simulink model "Drone_Response_v5"  (R2024b)
settings: Solver=VariableStepAuto  StartTime=0.0  StopTime=17.980265000000003  MaxStep=0.01  RelTol=1e-6  AbsTol=1e-8
model workspace (MAT data in the model file):
  Fx_gust = 1
  Fy_gust = 1
  Fz_gust = 0.5
  Ixx = 0.05
  Iyy = 0.05
  Izz = 0.1
  Kd_phi = 0.5
  Kd_psi = 0.12
  Kd_theta = 0.28
  Kd_x = 0.5
  Kd_y = 0.5
  Kd_z = 12
  Ki_phi = 0
  Ki_psi = 0
  Ki_theta = 0.28
  Ki_x = 0
  Ki_y = 0
  Ki_z = 0.1
  Kp_phi = 1
  Kp_psi = 0.012
  Kp_theta = 0.8
  Kp_x = 0.1
  Kp_y = 0.1
  Kp_z = 12
  N_phi = 100
  N_psi = 100
  N_theta = 100
  N_x = 100
  N_y = 100
  N_z = 100
  Tmax = 22.4649
  Tmin = 0
  d = 0.2
  disturbances_enabled = 0
  flight_mode = 3
  frozen_configuration : object (value not decoded)
  frozen_filter_init_184 = 0.000968325935072
  frozen_filter_init_244 = -0.00996407378017
  frozen_filter_init_247 = 0.0189310533866
  frozen_filter_init_63 = 0.120731046274
  frozen_filter_init_8 = -0.00230151225217
  frozen_filter_init_92 = -0.00686694318858
  g = 9.81
  inv_m = 0.333333333333
  kf = 4e-05
  km = 1e-06
  m = 3
  mg = 29.43
  omega_hover = 399.217985567
  omega_init = 428.879353665
  phi0 = 0.0109224523708
  phi_des = 0
  phi_dot0 = -0.0602280499979
  phi_manual = 0
  pitch_pair_allocation = 2.5
  psi0 = 2.78260847334
  psi_des = 0
  psi_dot0 = 0.0811475700195
  psi_hold = 0
  psi_manual = 0
  rad_to_deg = 57.2957795131
  replay_collective_to_pair_thrust_N = 58
  replay_enabled = 1
  replay_hover_collective = 0.24829455053
  replay_hover_pair_thrust_scale_N = 51.3503013771
  response_axis_nx = -0.0174524064373
  response_axis_ny = 0
  response_axis_nz = 0.999847695156
  response_experiment_status = 'Frozen experimental replay: ascent training8.7805; reserved descent2.6653; full airborne0. NOT a general8/10 release.'
  response_manual_enable : timeseries (value not decoded)
  response_v5_status = 'Experimental controller design; general8/10 not achieved; manufacturer cap provisional'
  response_vertical_drag_rate = 0.5
  roll_motor_allocation = 1.25
  rtl_accel_ff_gain = 0.856563645814
  rtl_altitude_accel_command : timeseries (value not decoded)
  rtl_altitude_command : timeseries (value not decoded)
  rtl_altitude_filter_init = 0.354897972076
  rtl_attitude_inputs : Simulink.SimulationData.Dataset (value not decoded)
  rtl_drag_rate = 1
  rtl_east_target : timeseries (value not decoded)
  rtl_north_target : timeseries (value not decoded)
  seed_phi = 104
  seed_psi = 106
  seed_theta = 105
  seed_x = 101
  seed_y = 102
  seed_z = 103
  sensor_noise_enabled = 0
  sensor_noise_tau_attitude = 0.1
  sensor_noise_tau_position = 0.2
  sensor_sample_time = 0.02
  sigma_phi = 0.000349065850399
  sigma_psi = 0.000872664625997
  sigma_theta = 0.000349065850399
  sigma_x = 0.002
  sigma_y = 0.002
  sigma_z = 0.001
  t_Fx_end = 11
  t_Fx_start = 10
  t_Fy_end = 16
  t_Fy_start = 15
  t_Fz_end = 21
  t_Fz_start = 20
  t_pitch_end = 30.5
  t_pitch_start = 30
  t_roll_end = 25.5
  t_roll_start = 25
  t_step_xy = 1
  t_step_yaw = 1
  t_step_z = 0
  t_stop = 17.980265
  t_yaw_end = 35.5
  t_yaw_start = 35
  tau_m = 0.02
  tau_pitch_gust = 0.01
  tau_roll_gust = 0.01
  tau_yaw_gust = 0.002
  theta0 = 0.0291618371461
  theta_des = 0.174532925199
  theta_dot0 = 0.0296232047334
  theta_manual = 0
  tilt_max = 0.1745
  visual_arm_length = 0.35
  visual_demo_disturbances = 1
  visual_demo_sensor_noise = 0
  visual_demo_stop_time = 60
  visual_demo_yaw = 0.523598775598
  visual_frame_rate = 30
  visual_playback_speed = 4
  visual_record_video = 0
  visual_trail_length = inf
  vx0 = 0.0296084290651
  vy0 = 0.0198878378966
  vz0 = 0.0507991741846
  x0 = 0
  x_des = 4
  x_hold = 0
  x_manual = 0
  y0 = 0
  y_des = 2
  y_hold = 0
  y_manual = 0
  yaw_motor_allocation = 10
  z0 = 0.367621053576
  z_des = 1
  z_hold = 1
  z_manual = 1
libraries: slpidlib x6
(part 2 of 2)

== system Drone_Response_v5/X_Position_Controller ==
  x_des : Inport
  x : Inport  Port=2
  Pitch_Command_Limit : Saturate  UpperLimit=tilt_max  LowerLimit=-tilt_max
  X_Position_Error : Sum  Inputs=+-|
  X_Position_PID : slpidlib/PID Controller  Controller=PID  Form=Parallel  TimeDomain=Continuous-time  UseExternalTs=off  SampleTime=-1  IntegratorMethod=Forward Euler  FilterMethod=Forward Euler  ControllerParametersSource=internal  P=Kp_x  I=Ki_x  UseKiTs=off  D=Kd_x  UseExternalDerivativeSource=off  N=N_x  UseFilter=on  TunerSelectOption=Transfer Function Based (PID Tuner App)  InitialConditionSource=internal  InitialConditionForIntegrator=0  InitialConditionForFilter=-0.000567351607968739  DifferentiatorICPrevScaledInput=0  ExternalReset=none  TrackingMode=off  Kt=1  LimitOutput=off  SatLimitsSource=internal  UpperSaturationLimit=inf  LowerSaturationLimit=-inf  LinearizeAsGain=on  AntiWindupMode=none  Kb=1  LimitIntegrator=off  UpperIntegratorSaturationLimit=inf  LowerIntegratorSaturationLimit=-inf  POutMin=[]  POutMax=[]  IOutMin=[]  IOutMax=[]  DOutMin=[]  DOutMax=[]  NOutMin=[]  NOutMax=[]  SumOutMin=[]  SumOutMax=[]  SaturationOutMin=[]  SaturationOutMax=[]  PParamMin=[]  PParamMax=[]  IParamMin=[]  IParamMax=[]  DParamMin=[]  DParamMax=[]  NParamMin=[]  NParamMax=[]  KbParamMin=[]  KbParamMax=[]  KtParamMin=[]  KtParamMax=[]  KbOutMin=[]  KbOutMax=[]  KtOutMin=[]  KtOutMax=[]  IntegratorOutMin=[]  IntegratorOutMax=[]  FilterOutMin=[]  FilterOutMax=[]  SumI1OutMin=[]  SumI1OutMax=[]  SumI2OutMin=[]  SumI2OutMax=[]  SumI3OutMin=[]  SumI3OutMax=[]  SumI4OutMin=[]  SumI4OutMax=[]  SumDOutMin=[]  SumDOutMax=[]  DifferentiatorOutMin=[]  DifferentiatorOutMax=[]  FilterDiffOutCoefMin=[]  FilterDiffOutCoefMax=[]  ReciprocalOutMin=[]  ReciprocalOutMax=[]  SumDenOutMin=[]  SumDenOutMax=[]  SumNumOutMin=[]  SumNumOutMax=[]  DivideOutMin=[]  DivideOutMax=[]  UdiffTsProdOutMin=[]  UdiffTsProdOutMax=[]  NTsProdOutMin=[]  NTsProdOutMax=[]  UintegralTsProdOutMin=[]  UintegralTsProdOutMax=[]  UngainTsProdOutMin=[]  UngainTsProdOutMax=[]  ClampingZeroOutDataTypeStr=Inherit: Inherit via back propagation  ClampingZeroOutMin=[]  ClampingZeroOutMax=[]  FilterDenConstantOutDataTypeStr=Inherit: Inherit via back propagation  FilterDenConstantOutMin=[]  FilterDenConstantOutMax=[]  PCopyOutDataTypeStr=Inherit: Inherit via back propagation  PCopyOutMin=[]  PCopyOutMax=[]  NCopyOutDataTypeStr=Inherit: Inherit via back propagation  NCopyOutMin=[]  NCopyOutMax=[]  IntegratorContinuousStateAttributes=''  IntegratorStateMustResolveToSignalObject=off  IntegratorRTWStateStorageClass=Auto  FilterContinuousStateAttributes=''  FilterStateMustResolveToSignalObject=off  FilterRTWStateStorageClass=Auto  ParallelPVariant=InternalParameters  IdealPVariant=Disabled  IVariant=InternalParameters  DVariant=InternalParameters  IntegratorVariant=Continuous  SatVariant=Disabled  AWVariant=Passthrough  PCopyVariant=Disabled  TRVariant=Disabled  FdbkBlocksVariant=Forward  IdealPFdbkVariant=Disabled  SatFdbkVariant=Disabled  DerivativeFilterVariant=ContFilter  NVariant=InternalParameters  NCopyVariant=Disabled  FilterICVariant=InternalICsFilter  IntegratorICVariant=InternalICs  ExternalResetVariant=Disabled  TRSumVariant=Passthrough  SumFdbkVariant=Disabled  SumVariant=Sum_PID  TsampFilterVariant=InternalTs  TsampNgainVariant=Passthrough  TsampIntegralVariant=Disabled_SignalSpec  ExternalSaturationOutDataTypeStr=Inherit: Same as second input  DerivativeSourceVariant=ErrorSignal  PreIntVariant=InternalPreInt
  theta_des : Outport
  wires:
  x_des/1 -> X_Position_Error/1
  X_Position_PID/1 -> Pitch_Command_Limit/1
  x/1 -> X_Position_Error/2
  X_Position_Error/1 -> X_Position_PID/1
  Pitch_Command_Limit/1 -> theta_des/1

== system Drone_Response_v5/Y_Position_Controller ==
  y : Inport
  y_des : Inport  Port=2
  Roll_Command_Limit : Saturate  UpperLimit=tilt_max  LowerLimit=-tilt_max
  Roll_Command_Sign : Gain  Gain=-1
  Y_Position_Error : Sum  Inputs=|-+
  Y_Position_PID : slpidlib/PID Controller  Controller=PID  Form=Parallel  TimeDomain=Continuous-time  UseExternalTs=off  SampleTime=-1  IntegratorMethod=Forward Euler  FilterMethod=Forward Euler  ControllerParametersSource=internal  P=Kp_y  I=Ki_y  UseKiTs=off  D=Kd_y  UseExternalDerivativeSource=off  N=N_y  UseFilter=on  TunerSelectOption=Transfer Function Based (PID Tuner App)  InitialConditionSource=internal  InitialConditionForIntegrator=0  InitialConditionForFilter=-0.000111447032045859  DifferentiatorICPrevScaledInput=0  ExternalReset=none  TrackingMode=off  Kt=1  LimitOutput=off  SatLimitsSource=internal  UpperSaturationLimit=inf  LowerSaturationLimit=-inf  LinearizeAsGain=on  AntiWindupMode=none  Kb=1  LimitIntegrator=off  UpperIntegratorSaturationLimit=inf  LowerIntegratorSaturationLimit=-inf  POutMin=[]  POutMax=[]  IOutMin=[]  IOutMax=[]  DOutMin=[]  DOutMax=[]  NOutMin=[]  NOutMax=[]  SumOutMin=[]  SumOutMax=[]  SaturationOutMin=[]  SaturationOutMax=[]  PParamMin=[]  PParamMax=[]  IParamMin=[]  IParamMax=[]  DParamMin=[]  DParamMax=[]  NParamMin=[]  NParamMax=[]  KbParamMin=[]  KbParamMax=[]  KtParamMin=[]  KtParamMax=[]  KbOutMin=[]  KbOutMax=[]  KtOutMin=[]  KtOutMax=[]  IntegratorOutMin=[]  IntegratorOutMax=[]  FilterOutMin=[]  FilterOutMax=[]  SumI1OutMin=[]  SumI1OutMax=[]  SumI2OutMin=[]  SumI2OutMax=[]  SumI3OutMin=[]  SumI3OutMax=[]  SumI4OutMin=[]  SumI4OutMax=[]  SumDOutMin=[]  SumDOutMax=[]  DifferentiatorOutMin=[]  DifferentiatorOutMax=[]  FilterDiffOutCoefMin=[]  FilterDiffOutCoefMax=[]  ReciprocalOutMin=[]  ReciprocalOutMax=[]  SumDenOutMin=[]  SumDenOutMax=[]  SumNumOutMin=[]  SumNumOutMax=[]  DivideOutMin=[]  DivideOutMax=[]  UdiffTsProdOutMin=[]  UdiffTsProdOutMax=[]  NTsProdOutMin=[]  NTsProdOutMax=[]  UintegralTsProdOutMin=[]  UintegralTsProdOutMax=[]  UngainTsProdOutMin=[]  UngainTsProdOutMax=[]  ClampingZeroOutDataTypeStr=Inherit: Inherit via back propagation  ClampingZeroOutMin=[]  ClampingZeroOutMax=[]  FilterDenConstantOutDataTypeStr=Inherit: Inherit via back propagation  FilterDenConstantOutMin=[]  FilterDenConstantOutMax=[]  PCopyOutDataTypeStr=Inherit: Inherit via back propagation  PCopyOutMin=[]  PCopyOutMax=[]  NCopyOutDataTypeStr=Inherit: Inherit via back propagation  NCopyOutMin=[]  NCopyOutMax=[]  IntegratorContinuousStateAttributes=''  IntegratorStateMustResolveToSignalObject=off  IntegratorRTWStateStorageClass=Auto  FilterContinuousStateAttributes=''  FilterStateMustResolveToSignalObject=off  FilterRTWStateStorageClass=Auto  ParallelPVariant=InternalParameters  IdealPVariant=Disabled  IVariant=InternalParameters  DVariant=InternalParameters  IntegratorVariant=Continuous  SatVariant=Disabled  AWVariant=Passthrough  PCopyVariant=Disabled  TRVariant=Disabled  FdbkBlocksVariant=Forward  IdealPFdbkVariant=Disabled  SatFdbkVariant=Disabled  DerivativeFilterVariant=ContFilter  NVariant=InternalParameters  NCopyVariant=Disabled  FilterICVariant=InternalICsFilter  IntegratorICVariant=InternalICs  ExternalResetVariant=Disabled  TRSumVariant=Passthrough  SumFdbkVariant=Disabled  SumVariant=Sum_PID  TsampFilterVariant=InternalTs  TsampNgainVariant=Passthrough  TsampIntegralVariant=Disabled_SignalSpec  ExternalSaturationOutDataTypeStr=Inherit: Same as second input  DerivativeSourceVariant=ErrorSignal  PreIntVariant=InternalPreInt
  phi_des : Outport
  wires:
  y/1 -> Y_Position_Error/1
  Y_Position_Error/1 -> Y_Position_PID/1
  y_des/1 -> Y_Position_Error/2
  Roll_Command_Sign/1 -> Roll_Command_Limit/1
  Y_Position_PID/1 -> Roll_Command_Sign/1
  Roll_Command_Limit/1 -> phi_des/1

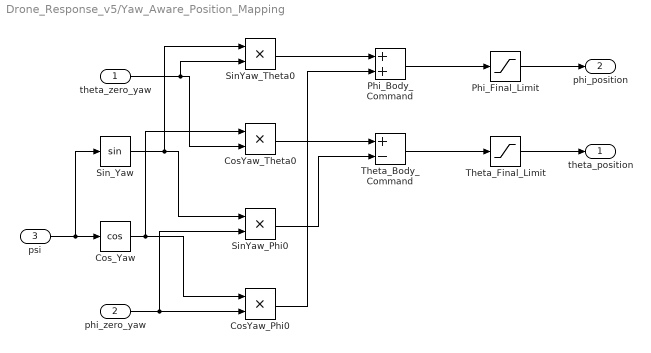
== system Drone_Response_v5/Yaw_Aware_Position_Mapping ==
  theta_zero_yaw : Inport
  phi_zero_yaw : Inport  Port=2
  psi : Inport  Port=3
  CosYaw_Phi0 : Product  Inputs=**
  CosYaw_Theta0 : Product  Inputs=**
  Cos_Yaw : Trigonometry  Operator=cos
  Phi_Body_Command : Sum
  Phi_Final_Limit : Saturate  UpperLimit=tilt_max  LowerLimit=-tilt_max
  SinYaw_Phi0 : Product  Inputs=**
  SinYaw_Theta0 : Product  Inputs=**
  Sin_Yaw : Trigonometry
  Theta_Body_Command : Sum  Inputs=+-
  Theta_Final_Limit : Saturate  UpperLimit=tilt_max  LowerLimit=-tilt_max
  theta_position : Outport
  phi_position : Outport  Port=2
  wires:
  Phi_Final_Limit/1 -> phi_position/1
  Phi_Body_Command/1 -> Phi_Final_Limit/1
  CosYaw_Phi0/1 -> Phi_Body_Command/2
  SinYaw_Theta0/1 -> Phi_Body_Command/1
  Theta_Final_Limit/1 -> theta_position/1
  Theta_Body_Command/1 -> Theta_Final_Limit/1
  SinYaw_Phi0/1 -> Theta_Body_Command/2
  CosYaw_Theta0/1 -> Theta_Body_Command/1
  phi_zero_yaw/1 -> SinYaw_Phi0/2, CosYaw_Phi0/2
  Sin_Yaw/1 -> SinYaw_Phi0/1, SinYaw_Theta0/1
  theta_zero_yaw/1 -> CosYaw_Theta0/2, SinYaw_Theta0/2
  Cos_Yaw/1 -> CosYaw_Theta0/1, CosYaw_Phi0/1
  psi/1 -> Cos_Yaw/1, Sin_Yaw/1

== system Drone_Response_v5/Yaw_Controller ==
  psi_des : Inport
  psi : Inport  Port=2
  Yaw_Error : Sum  Inputs=-+|
  Yaw_Motor_Allocation : Gain  Gain=yaw_motor_allocation
  Yaw_PID : slpidlib/PID Controller  Controller=PID  Form=Parallel  TimeDomain=Continuous-time  UseExternalTs=off  SampleTime=-1  IntegratorMethod=Forward Euler  FilterMethod=Forward Euler  ControllerParametersSource=internal  P=Kp_psi  I=Ki_psi  UseKiTs=off  D=Kd_psi  UseExternalDerivativeSource=off  N=N_psi  UseFilter=on  TunerSelectOption=Transfer Function Based (PID Tuner App)  InitialConditionSource=internal  InitialConditionForIntegrator=0  InitialConditionForFilter=-0.00860864472359648  DifferentiatorICPrevScaledInput=0  ExternalReset=none  TrackingMode=off  Kt=1  LimitOutput=off  SatLimitsSource=internal  UpperSaturationLimit=inf  LowerSaturationLimit=-inf  LinearizeAsGain=on  AntiWindupMode=none  Kb=1  LimitIntegrator=off  UpperIntegratorSaturationLimit=inf  LowerIntegratorSaturationLimit=-inf  POutMin=[]  POutMax=[]  IOutMin=[]  IOutMax=[]  DOutMin=[]  DOutMax=[]  NOutMin=[]  NOutMax=[]  SumOutMin=[]  SumOutMax=[]  SaturationOutMin=[]  SaturationOutMax=[]  PParamMin=[]  PParamMax=[]  IParamMin=[]  IParamMax=[]  DParamMin=[]  DParamMax=[]  NParamMin=[]  NParamMax=[]  KbParamMin=[]  KbParamMax=[]  KtParamMin=[]  KtParamMax=[]  KbOutMin=[]  KbOutMax=[]  KtOutMin=[]  KtOutMax=[]  IntegratorOutMin=[]  IntegratorOutMax=[]  FilterOutMin=[]  FilterOutMax=[]  SumI1OutMin=[]  SumI1OutMax=[]  SumI2OutMin=[]  SumI2OutMax=[]  SumI3OutMin=[]  SumI3OutMax=[]  SumI4OutMin=[]  SumI4OutMax=[]  SumDOutMin=[]  SumDOutMax=[]  DifferentiatorOutMin=[]  DifferentiatorOutMax=[]  FilterDiffOutCoefMin=[]  FilterDiffOutCoefMax=[]  ReciprocalOutMin=[]  ReciprocalOutMax=[]  SumDenOutMin=[]  SumDenOutMax=[]  SumNumOutMin=[]  SumNumOutMax=[]  DivideOutMin=[]  DivideOutMax=[]  UdiffTsProdOutMin=[]  UdiffTsProdOutMax=[]  NTsProdOutMin=[]  NTsProdOutMax=[]  UintegralTsProdOutMin=[]  UintegralTsProdOutMax=[]  UngainTsProdOutMin=[]  UngainTsProdOutMax=[]  ClampingZeroOutDataTypeStr=Inherit: Inherit via back propagation  ClampingZeroOutMin=[]  ClampingZeroOutMax=[]  FilterDenConstantOutDataTypeStr=Inherit: Inherit via back propagation  FilterDenConstantOutMin=[]  FilterDenConstantOutMax=[]  PCopyOutDataTypeStr=Inherit: Inherit via back propagation  PCopyOutMin=[]  PCopyOutMax=[]  NCopyOutDataTypeStr=Inherit: Inherit via back propagation  NCopyOutMin=[]  NCopyOutMax=[]  IntegratorContinuousStateAttributes=''  IntegratorStateMustResolveToSignalObject=off  IntegratorRTWStateStorageClass=Auto  FilterContinuousStateAttributes=''  FilterStateMustResolveToSignalObject=off  FilterRTWStateStorageClass=Auto  ParallelPVariant=InternalParameters  IdealPVariant=Disabled  IVariant=InternalParameters  DVariant=InternalParameters  IntegratorVariant=Continuous  SatVariant=Disabled  AWVariant=Passthrough  PCopyVariant=Disabled  TRVariant=Disabled  FdbkBlocksVariant=Forward  IdealPFdbkVariant=Disabled  SatFdbkVariant=Disabled  DerivativeFilterVariant=ContFilter  NVariant=InternalParameters  NCopyVariant=Disabled  FilterICVariant=InternalICsFilter  IntegratorICVariant=InternalICs  ExternalResetVariant=Disabled  TRSumVariant=Passthrough  SumFdbkVariant=Disabled  SumVariant=Sum_PID  TsampFilterVariant=InternalTs  TsampNgainVariant=Passthrough  TsampIntegralVariant=Disabled_SignalSpec  ExternalSaturationOutDataTypeStr=Inherit: Same as second input  DerivativeSourceVariant=ErrorSignal  PreIntVariant=InternalPreInt
  Yaw_cmd : Outport
  wires:
  Yaw_PID/1 -> Yaw_Motor_Allocation/1
  Yaw_Error/1 -> Yaw_PID/1
  psi/1 -> Yaw_Error/1
  psi_des/1 -> Yaw_Error/2
  Yaw_Motor_Allocation/1 -> Yaw_cmd/1

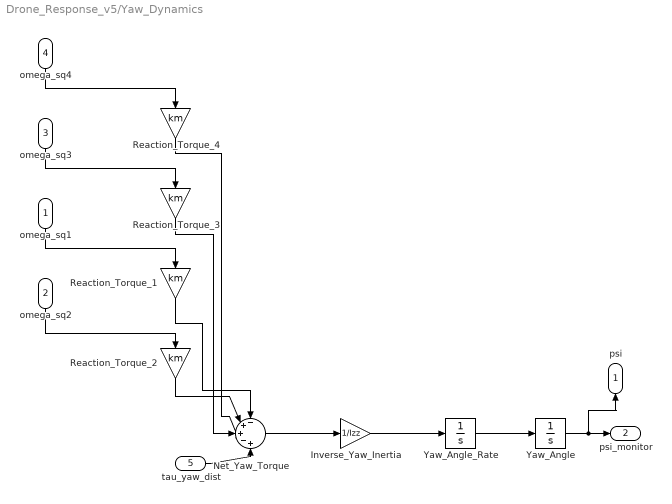
== system Drone_Response_v5/Yaw_Dynamics ==
  omega_sq1 : Inport
  omega_sq2 : Inport  Port=2
  omega_sq3 : Inport  Port=3
  omega_sq4 : Inport  Port=4
  tau_yaw_dist : Inport  Port=5
  Inverse_Yaw_Inertia : Gain  Gain=1/Izz
  Net_Yaw_Torque : Sum  Inputs=-++-+
  Reaction_Torque_{1..4} (4 alike) : Gain  Gain=km
  Yaw_Angle : Integrator  InitialCondition=psi0
  Yaw_Angle_Rate : Integrator  InitialCondition=psi_dot0
  psi : Outport
  psi_monitor : Outport  Port=2
  wires:
  Reaction_Torque_2/1 -> Net_Yaw_Torque/2
  omega_sq2/1 -> Reaction_Torque_2/1
  Reaction_Torque_4/1 -> Net_Yaw_Torque/4
  omega_sq1/1 -> Reaction_Torque_1/1
  omega_sq3/1 -> Reaction_Torque_3/1
  omega_sq4/1 -> Reaction_Torque_4/1
  Reaction_Torque_1/1 -> Net_Yaw_Torque/1
  Reaction_Torque_3/1 -> Net_Yaw_Torque/3
  Net_Yaw_Torque/1 -> Inverse_Yaw_Inertia/1
  Inverse_Yaw_Inertia/1 -> Yaw_Angle_Rate/1
  Yaw_Angle_Rate/1 -> Yaw_Angle/1
  Yaw_Angle/1 -> psi/1, psi_monitor/1
  tau_yaw_dist/1 -> Net_Yaw_Torque/5
